simulink model "TD"  (R2016b)
settings: Solver=VariableStepAuto  StartTime=0.0  StopTime=50  RelTol=1e-3
libraries: simulink x1
settings Model: Creator=lenovo  LastModifiedBy=lenovo

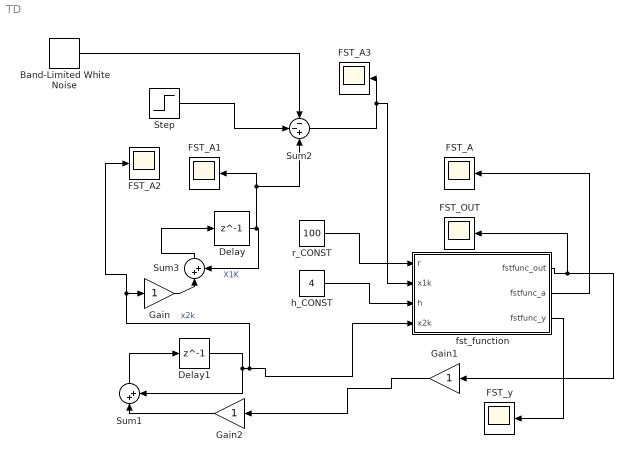
== system TD ==
  Band-Limited White Noise : simulink/Sources/Band-Limited White Noise  Cov=[0.1]  Ts=0.1  seed=[23341]
  Delay : Delay  DelayLength=1  InitialCondition=0
  Delay1 : Delay  DelayLength=1
  FST_A{,1..3} (4 alike) : Scope
  FST_OUT : Scope
  FST_y : Scope
  Gain : Gain
  Gain1 : Gain
  Gain2 : Gain
  Step : Step  Time=0  After=10  SampleTime=0
  Sum1 : Sum  Inputs=|++
  Sum2 : Sum  Inputs=--+
  Sum3 : Sum  Inputs=|++
  fst_function : Subsystem
  h_CONST : Constant  Value=4
  r_CONST : Constant  Value=100
  wires:
  Delay/1 -> Sum2/3, FST_A1/1, Sum3/2  "X1K"
  Delay1/1 -> Sum1/2, Gain/1, FST_A2/1, fst_function/4(x2k)  "x2k"
  fst_function/1(fstfunc_out) -> Gain1/1, FST_OUT/1
  r_CONST/1 -> fst_function/1(r)
  Sum2/1 -> FST_A3/1, fst_function/2(x1k)
  h_CONST/1 -> fst_function/3(h)
  fst_function/2(fstfunc_a) -> FST_A/1
  fst_function/3(fstfunc_y) -> FST_y/1
  Gain/1 -> Sum3/1
  Sum3/1 -> Delay/1
  Gain1/1 -> Gain2/1
  Sum1/1 -> Delay1/1
  Gain2/1 -> Sum1/1
  Step/1 -> Sum2/2
  Band-Limited White Noise/1 -> Sum2/1

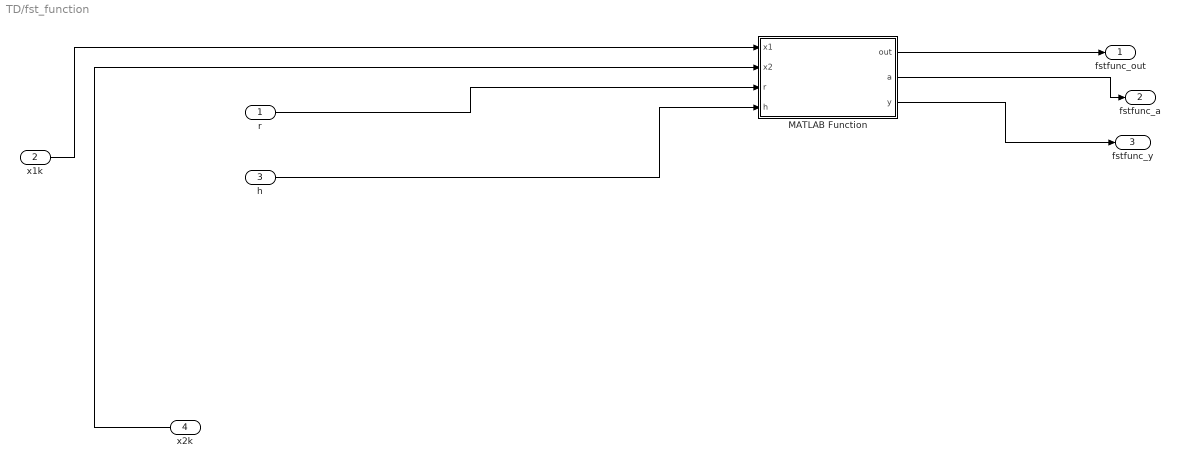
== system TD/fst_function ==
  r : Inport
  x1k : Inport  Port=2
  h : Inport  Port=3
  x2k : Inport  Port=4
  MATLAB Function : MATLAB Function  TreatAsAtomicUnit=on
  fstfunc_out : Outport
  fstfunc_a : Outport  Port=2
  fstfunc_y : Outport  Port=3
  wires:
  x2k/1 -> MATLAB Function/2(x2)
  r/1 -> MATLAB Function/3(r)
  h/1 -> MATLAB Function/4(h)
  MATLAB Function/1(out) -> fstfunc_out/1
  x1k/1 -> MATLAB Function/1(x1)
  MATLAB Function/2(a) -> fstfunc_a/1
  MATLAB Function/3(y) -> fstfunc_y/1

== matlab function TD/fst_function/MATLAB Function ==
  data: x1 input; out output; x2 input; r input; h input; a output; y output
function [out,a,y] = fst_test(x1,x2,r,h)
d=r*h;
d0=d*h;
y=x1+h*x2;
a0=sqrt(d*d+8*r*abs(y));
absy=abs(y);
if absy>d0
    a=x2+0.5*a0-0.5*d;
else
    a=x2+y/h;
end
absa=abs(a);
if absa<=d0
    out=-r*a/d;
else
    out=-r*sign(a);
end

end
